simulink model "PhaseToTimeRefMod"  (R2016b)
settings: Solver=VariableStepAuto  StartTime=0.0  StopTime=10.0  RelTol=1e-3
settings Model: DataDictionary=DataDictionary.sldd  Creator=lucadelaat  LastModifiedBy=Taeke

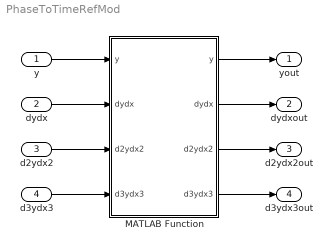
== system PhaseToTimeRefMod ==
  y : Inport  PortDimensions=numberSamplePoints  BusOutputAsStruct=on
  dydx : Inport  Port=2  PortDimensions=numberSamplePoints  BusOutputAsStruct=on
  d2ydx2 : Inport  Port=3  PortDimensions=numberSamplePoints  BusOutputAsStruct=on
  d3ydx3 : Inport  Port=4  PortDimensions=numberSamplePoints  BusOutputAsStruct=on
  MATLAB Function : MATLAB Function  TreatAsAtomicUnit=on
  yout : Outport  PortDimensions=numberSamplePoints
  dydxout : Outport  Port=2  PortDimensions=numberSamplePoints
  d2ydx2out : Outport  Port=3  PortDimensions=numberSamplePoints
  d3ydx3out : Outport  Port=4  PortDimensions=numberSamplePoints
  wires:
  y/1 -> MATLAB Function/1("y ")
  dydx/1 -> MATLAB Function/2("dydx ")
  d2ydx2/1 -> MATLAB Function/3("d2ydx2 ")
  d3ydx3/1 -> MATLAB Function/4("d3ydx3 ")
  MATLAB Function/1(y) -> yout/1
  MATLAB Function/2(dydx) -> dydxout/1
  MATLAB Function/3(d2ydx2) -> d2ydx2out/1
  MATLAB Function/4(d3ydx3) -> d3ydx3out/1

== matlab function PhaseToTimeRefMod/MATLAB Function ==
  data: y input; y output; dydx input; d2ydx2 input; d3ydx3 input; dydx output; d2ydx2 output; d3ydx3 output
function [y, dydx, d2ydx2, d3ydx3] = timeToPhase(y, dydx, d2ydx2, d3ydx3)
%Defivatives are genrated for %, we want to convert this into time
%100% stride = 2 steps
%if step frequency is 1 this means 100 [%] stride is 2 [s]
converter = 100/4; %[%/s]

y      = y;
dydx   = converter * dydx;
d2ydx2 = converter^2 * d2ydx2;
d3ydx3 = converter^3 * d3ydx3;
end
